simulink model "Twelve_quad_formation_301114"  (R2012b)
settings: Solver=ode5  StartTime=0.0  StopTime=inf  FixedStep=sample_time  RelTol=1e-3
InitFcn:
  | sample_time=0.005;%0.004;%0.0025;%0.02;
  | sample_time_Vicon = 0.005;
  | DeltaT = 0.02;
  | g = 9.81;
  | H0 = g%0.3165;
  | Kl = 1;
  | 
  | Q6_mass = 0.8;
  | 
  | Q6_Omega_r = 1.2; %for horizon ref
  | Q6_Zeta_r = 0.707; %for horizon ref
  | Q6_Omega_r_h = 2;%for vertical ref
  | Q6_Zeta_r_h = 0.7; %for vertical ref
  | 
  | 
  | Q6_Omega = 1.5; %for horizon control
  | Q6_Zeta = 0.507; %for horizon control
  | Q6_Omega_h= 2 %for vertical control
  | Q6_Zeta_h = 0.5; %for vertical control
  | 
  | 
  | Q6_acc_max = 5;%horizontal max acc
  | Q6_acc_max_h = 5;%horizontal max acc
  | 
  | omega_circle = 10*pi/180;
  | 
  | omega_h = 0.1;%Ascending speed
  | PI = pi;
  | Circle_R = 2;
  | 
  | 
  | MAX_Height = -2;
  | 
  | 
  | % for NN
  | n = 5;
  | r = 3;
  | n2 = 5;
  | NN_ST = 0.02;
  | 
  | GAMA_V = 6;
  | gama_V_e = 0.01;
  | 
  | GAMA_W = GAMA_V;
  | gama_W_e =0.01;
  | 
  | % deadzone
  | NN_Deadzone_Z = 0;
  | 
  | % inputs nomalizaton parameters
  | NN_Z_y_min = -3;
  | NN_Z_y_max = 0.5;
  | 
  | NN_Z_v_max = 8;
  | NN_Z_v_min = -NN_Z_v_max;
  | 
  | % alpha = 0.034;
  | alpha = 1;
  | % c_f = 0.0015;
  | c_f = 0.001;
  | ... (+1 lines)
libraries: X330_Control x60, simulink x24
(part 3 of 3)

== system Twelve_quad_formation_301114/Vicon_Data/Process Vicon Raw Data and Filter 8/Flip_pi1/Flip_0_to_2pi/Flip_2pi ==
  Angle : Inport
  Bias : Bias  Bias=-2*pi
  Constant : Constant  Value=2*pi
  Data Type Duplicate : DataTypeDuplicate
  Modulo : Math  Operator=mod  SaturateOnIntegerOverflow=on
  Sign1 : Signum
  Switch : Switch
  Angle_Flip : Outport
  wires:
  Angle/1 -> Modulo/1, Sign1/1, Data Type Duplicate/1
  Constant/1 -> Modulo/2
  Modulo/1 -> Bias/1, Switch/1
  Sign1/1 -> Switch/2
  Bias/1 -> Switch/3
  Switch/1 -> Angle_Flip/1, Data Type Duplicate/2

== system Twelve_quad_formation_301114/Vicon_Data/Process Vicon Raw Data and Filter 9/Flip_pi1/Flip_0_to_2pi/Flip_2pi ==
  Angle : Inport
  Bias : Bias  Bias=-2*pi
  Constant : Constant  Value=2*pi
  Data Type Duplicate : DataTypeDuplicate
  Modulo : Math  Operator=mod  SaturateOnIntegerOverflow=on
  Sign1 : Signum
  Switch : Switch
  Angle_Flip : Outport
  wires:
  Switch/1 -> Data Type Duplicate/2, Angle_Flip/1
  Bias/1 -> Switch/3
  Sign1/1 -> Switch/2
  Modulo/1 -> Switch/1, Bias/1
  Constant/1 -> Modulo/2
  Angle/1 -> Data Type Duplicate/1, Sign1/1, Modulo/1

== stateflow chart Twelve_quad_formation_301114/Subsystem/Trajectory Logic/ SF ==
  state Airborne
    state Stage6
      state Red_UAV1 [parallel]
        du:PosDes_UAV1[0] = (-1.457 - PosDes_UAV1[0])*0.5*DeltaT + PosDes_UAV1[0];
        PosDes_UAV1[1] = (1.457 - PosDes_UAV1[1])*0.5*DeltaT + PosDes_UAV1[1] ;
        PosDes_UAV1[2] = -1.2;
        settings: executionOrder=1
      state PWM1 [parallel]
        du:    Increm = Increm + DeltaT
        settings: executionOrder=2
      state Green_UAV2 [parallel]
        du:PosDes_UAV2[0] =(1.457 - PosDes_UAV2[0])*0.5*DeltaT + PosDes_UAV2[0] ;
        PosDes_UAV2[1] = (1.457 - PosDes_UAV2[1])*0.5*DeltaT + PosDes_UAV2[1];
        PosDes_UAV2[2] = -1.2;
        settings: executionOrder=3
      state Blue_UAV3 [parallel]
        du:PosDes_UAV3[0] = (-1.457 - PosDes_UAV3[0])*0.5*DeltaT + PosDes_UAV3[0] ;
        PosDes_UAV3[1] = (-1.457 - PosDes_UAV3[1])*0.5*DeltaT + PosDes_UAV3[1];
        PosDes_UAV3[2] = -1.2;
        settings: executionOrder=4
      state Purple_UAV4 [parallel]
        du:PosDes_UAV4[0] = (1.457 - PosDes_UAV4[0])*0.5*DeltaT + PosDes_UAV4[0];
        PosDes_UAV4[1] = (-1.457 - PosDes_UAV4[1])*0.5*DeltaT + PosDes_UAV4[1];
        PosDes_UAV4[2] = -1.2;
        settings: executionOrder=5
    state TakeOff
      du:		HoverThrottle = (H0 - HoverThrottle)*2*DeltaT + HoverThrottle ;
      PosDes_UAV1[2] = (-1.2 - PosDes_UAV1[2])*1*DeltaT + PosDes_UAV1[2] ; PosDes_UAV7[2] = (-1.2 - PosDes_UAV7[2])*1*DeltaT + PosDes_UAV7[2] ;
      PosDes_UAV2[2] = (-1.2 - PosDes_UAV2[2])*1*DeltaT + PosDes_UAV2[2] ; PosDes_UAV8[2] = (-1.2 - PosDes_UAV8[2])*1*DeltaT + PosDes_UAV8[2] ;
      PosDes_UAV3[2] = (-1.2 - PosDes_UAV3[2])*1*DeltaT + PosDes_UAV3[2] ; PosDes_UAV9[2] = (-1.2 - PosDes_UAV9[2])*1*DeltaT + PosDes_UAV9[2] ;
      PosDes_UAV4[2] = (-1.2 - PosDes_UAV4[2])*1*DeltaT + PosDes_UAV4[2] ; PosDes_UAV10[2] = (-1.2 - PosDes_UAV10[2])*1*DeltaT + PosDes_UAV10[2] ;
      PosDes_UAV5[2] = (-1.2 - PosDes_UAV5[2])*1*DeltaT + PosDes_UAV5[2] ; PosDes_UAV11[2] = (-1.2 - PosDes_UAV11[2])*1*DeltaT + PosDes_UAV11[2] ;
      PosDes_UAV6[2] = (-1.2 - PosDes_UAV6[2])*1*DeltaT + PosDes_UAV6[2] ; PosDes_UAV12[2] = (-1.2 - PosDes_UAV12[2])*1*DeltaT + PosDes_UAV12[2] ;
    state Stage1
      state Purple_UAV7 [parallel]
        du:PosDes_UAV7[0] = (3-PosDes_UAV7[0])*0.75*DeltaT + PosDes_UAV7[0];
        PosDes_UAV7[1] = (-1-PosDes_UAV7[1])*0.75*DeltaT+PosDes_UAV7[1];
        PosDes_UAV7[2] = (-1.2-PosDes_UAV7[2])*0.75*DeltaT+PosDes_UAV7[2];
        settings: executionOrder=1
      state Red_UAV1 [parallel]
        du:PosDes_UAV1[0] = (3- PosDes_UAV1[0])*0.75*DeltaT + PosDes_UAV1[0] ;
        PosDes_UAV1[1] = (3- PosDes_UAV1[1])*0.75*DeltaT + PosDes_UAV1[1] ;
        PosDes_UAV1[2] = (-1.2- PosDes_UAV1[2])*0.75*DeltaT + PosDes_UAV1[2] ;
        settings: executionOrder=2
      state Purple_UAV8 [parallel]
        du:PosDes_UAV8[0] = (-3-PosDes_UAV8[0])*0.75*DeltaT + PosDes_UAV8[0];
        PosDes_UAV8[1] = (-1-PosDes_UAV8[1])*0.75*DeltaT+PosDes_UAV8[1];
        PosDes_UAV8[2] = (-1.2-PosDes_UAV8[2])*0.75*DeltaT+PosDes_UAV8[2];
        settings: executionOrder=3
      state Green_UAV2 [parallel]
        du:PosDes_UAV2[0] = (-3-PosDes_UAV2[0])*0.75*DeltaT+PosDes_UAV2[0];
        PosDes_UAV2[1] = (3-PosDes_UAV2[1])*0.75*DeltaT+PosDes_UAV2[1];
        PosDes_UAV2[2] = (-1.2-PosDes_UAV2[2])*0.75*DeltaT+PosDes_UAV2[2];
        settings: executionOrder=4
      state Blue_UAV3 [parallel]
        du:PosDes_UAV3[0] = (3-PosDes_UAV3[0])*0.75*DeltaT + PosDes_UAV3[0];
        PosDes_UAV3[1] = (2-PosDes_UAV3[1])*0.75*DeltaT+PosDes_UAV3[1];
        PosDes_UAV3[2] = (-1.2-PosDes_UAV3[2])*0.75*DeltaT+PosDes_UAV3[2];
        settings: executionOrder=5
      state Purple_UAV9 [parallel]
        du:PosDes_UAV9[0] = (3-PosDes_UAV9[0])*0.75*DeltaT + PosDes_UAV9[0];
        PosDes_UAV9[1] = (-2-PosDes_UAV9[1])*0.75*DeltaT+PosDes_UAV9[1];
        PosDes_UAV9[2] = (-1.2-PosDes_UAV9[2])*0.75*DeltaT+PosDes_UAV9[2];
        settings: executionOrder=6
      state Purple_UAV4 [parallel]
        du:PosDes_UAV4[0] = (-3-PosDes_UAV4[0])*0.75*DeltaT + PosDes_UAV4[0];
        PosDes_UAV4[1] = (2-PosDes_UAV4[1])*0.75*DeltaT+PosDes_UAV4[1];
        PosDes_UAV4[2] = (-1.2-PosDes_UAV4[2])*0.75*DeltaT+PosDes_UAV4[2];
        settings: executionOrder=7
      state Purple_UAV12 [parallel]
        du:PosDes_UAV10[0] = (-3-PosDes_UAV10[0])*0.75*DeltaT + PosDes_UAV10[0];
        PosDes_UAV10[1] = (-2-PosDes_UAV10[1])*0.75*DeltaT+PosDes_UAV10[1];
        PosDes_UAV10[2] = (-1.2-PosDes_UAV10[2])*0.75*DeltaT+PosDes_UAV10[2];
        settings: executionOrder=8
      state Purple_UAV5 [parallel]
        du:PosDes_UAV5[0] = (3-PosDes_UAV5[0])*0.75*DeltaT + PosDes_UAV5[0];
        PosDes_UAV5[1] = (1-PosDes_UAV5[1])*0.75*DeltaT+PosDes_UAV5[1];
        PosDes_UAV5[2] = (-1.2-PosDes_UAV5[2])*0.75*DeltaT+PosDes_UAV5[2];
        settings: executionOrder=9
      state Purple_UAV11 [parallel]
        du:PosDes_UAV11[0] = (3-PosDes_UAV11[0])*0.75*DeltaT + PosDes_UAV11[0];
        PosDes_UAV11[1] = (-3-PosDes_UAV11[1])*0.75*DeltaT+PosDes_UAV11[1];
        PosDes_UAV11[2] = (-1.2-PosDes_UAV11[2])*0.75*DeltaT+PosDes_UAV11[2];
        settings: executionOrder=10
      state Purple_UAV6 [parallel]
        du:PosDes_UAV6[0] = (-3-PosDes_UAV6[0])*0.75*DeltaT + PosDes_UAV6[0];
        PosDes_UAV6[1] = (1-PosDes_UAV6[1])*0.75*DeltaT+PosDes_UAV6[1];
        PosDes_UAV6[2] = (-1.2-PosDes_UAV6[2])*0.75*DeltaT+PosDes_UAV6[2];
        settings: executionOrder=11
      state Purple_UAV10 [parallel]
        du:PosDes_UAV4[0] = (-3-PosDes_UAV4[0])*0.75*DeltaT + PosDes_UAV4[0];
        PosDes_UAV4[1] = (-3-PosDes_UAV4[1])*0.75*DeltaT+PosDes_UAV4[1];
        PosDes_UAV4[2] = (-1.2-PosDes_UAV4[2])*0.75*DeltaT+PosDes_UAV4[2];
        settings: executionOrder=12
    state Stage7
      state Red_UAV1 [parallel]
        du:PosDes_UAV1[0] = 3.5*cos(81.087*PI/180-Increm*omega_circle)-2;
        PosDes_UAV1[1] = 3.5*sin(81.087*PI/180-Increm*omega_circle)-2 ;
        PosDes_UAV1[2] = -1.2;
        settings: executionOrder=1
      state PWM1 [parallel]
        du:    Increm = Increm + DeltaT
        settings: executionOrder=2
      state Green_UAV2 [parallel]
        du:PosDes_UAV2[0] = 3.5*cos(351.087*PI/180-Increm*omega_circle)-2;
        PosDes_UAV2[1] = 3.5*sin(351.087*PI/180-Increm*omega_circle)+2;
        PosDes_UAV2[2] = -1.2;
        settings: executionOrder=3
      state Blue_UAV3 [parallel]
        du:PosDes_UAV3[0] = 3.5*cos(171.087*PI/180-Increm*omega_circle)+2  ;
        PosDes_UAV3[1] = 3.5*sin(171.087*PI/180-Increm*omega_circle)-2;
        PosDes_UAV3[2] = -1.2;
        settings: executionOrder=4
      state Purple_UAV4 [parallel]
        du:PosDes_UAV4[0] = 3.5*cos(261.087*PI/180-Increm*omega_circle)+2 ;
        PosDes_UAV4[1] = 3.5*sin(261.087*PI/180-Increm*omega_circle)+2;
        PosDes_UAV4[2] = -1.2;
        settings: executionOrder=5
    state Stage2
      state Red_UAV1 [parallel]
        du:PosDes_UAV1[0] = (0.8 - PosDes_UAV1[0])*0.5*DeltaT + PosDes_UAV1[0]  ;
        PosDes_UAV1[1] = (2 - PosDes_UAV1[1])*0.5*DeltaT + PosDes_UAV1[1]  ;
        PosDes_UAV1[2] = -1.2 ;
        settings: executionOrder=1
      state PWM2 [parallel]
        du:    Increm = Increm + DeltaT
        settings: executionOrder=2
      state Green_UAV2 [parallel]
        du:PosDes_UAV2[0] = (-0.8 - PosDes_UAV2[0])*0.5*DeltaT + PosDes_UAV2[0];
        PosDes_UAV2[1] = (2 - PosDes_UAV2[1])*0.5*DeltaT + PosDes_UAV2[1];
        PosDes_UAV2[2] = -1.2;
        settings: executionOrder=3
      state Blue_UAV3 [parallel]
        du:PosDes_UAV3[0] = (0.8 - PosDes_UAV3[0])*0.5*DeltaT + PosDes_UAV3[0];
        PosDes_UAV3[1] = (-2 - PosDes_UAV3[1])*0.5*DeltaT + PosDes_UAV3[1];
        PosDes_UAV3[2] = -1.2;
        settings: executionOrder=4
      state Purple_UAV4 [parallel]
        du:PosDes_UAV4[0] = (-0.8 - PosDes_UAV4[0])*0.5*DeltaT + PosDes_UAV4[0];
        PosDes_UAV4[1] = (-2 - PosDes_UAV4[1])*0.5*DeltaT + PosDes_UAV4[1];
        PosDes_UAV4[2] = -1.2;
        settings: executionOrder=5
    state Stage8
      state Red_UAV1 [parallel]
        du:PosDes_UAV1[0] = (2 - PosDes_UAV1[0])*0.5*DeltaT + PosDes_UAV1[0];
        PosDes_UAV1[1] = (-2 - PosDes_UAV1[1])*0.5*DeltaT + PosDes_UAV1[1];
        PosDes_UAV1[2] = -1.2;
        settings: executionOrder=1
      state PWM1 [parallel]
        du:    Increm = Increm + DeltaT
        settings: executionOrder=2
      state Green_UAV2 [parallel]
        du:PosDes_UAV2[0] = (-2 - PosDes_UAV2[0])*0.5*DeltaT + PosDes_UAV2[0];
        PosDes_UAV2[1] = (-2 - PosDes_UAV2[1])*0.5*DeltaT + PosDes_UAV2[1];
        PosDes_UAV2[2] = -1.2;
        settings: executionOrder=3
      state Blue_UAV3 [parallel]
        du:PosDes_UAV3[0] = (2 - PosDes_UAV3[0])*0.5*DeltaT + PosDes_UAV3[0] ;
        PosDes_UAV3[1] = (2 - PosDes_UAV3[1])*0.5*DeltaT + PosDes_UAV3[1];
        PosDes_UAV3[2] = -1.2;
        settings: executionOrder=4
      state Purple_UAV4 [parallel]
        du:PosDes_UAV4[0] = (-2 - PosDes_UAV4[0])*0.5*DeltaT + PosDes_UAV4[0];
        PosDes_UAV4[1] = (2 - PosDes_UAV4[1])*0.5*DeltaT + PosDes_UAV4[1];
        PosDes_UAV4[2] = -1.2;
        settings: executionOrder=5
    state Stage3
      state Red_UAV1 [parallel]
        du:PosDes_UAV1[0] = 0.8-Increm;
        PosDes_UAV1[1] = 0.625*(0.8-Increm)*(0.8-Increm)+1.6 ;
        PosDes_UAV1[2] = -1.2;
        settings: executionOrder=1
      state PWM1 [parallel]
        du:    Increm = Increm + DeltaT
        settings: executionOrder=2
      state Green_UAV2 [parallel]
        du:PosDes_UAV2[0] = -0.8+Increm;
        PosDes_UAV2[1] = -0.625*(0.8-Increm)*(0.8-Increm)+2.4;
        PosDes_UAV2[2] = -1.2;
        settings: executionOrder=3
      state Blue_UAV3 [parallel]
        du:PosDes_UAV3[0] = 0.8 - Increm;
        PosDes_UAV3[1] = 0.625*(0.8-Increm)*(0.8-Increm)-2.4;
        PosDes_UAV3[2] = -1.2;
        settings: executionOrder=4
      state Purple_UAV4 [parallel]
        du:PosDes_UAV4[0] = -0.8 + Increm;
        PosDes_UAV4[1] = -0.625*(0.8-Increm)*(0.8-Increm)-1.6;
        PosDes_UAV4[2] = -1.2;
        settings: executionOrder=5
    state Stage9
      state Red_UAV1 [parallel]
        du:PosDes_UAV1[0] = (0 - PosDes_UAV1[0])*0.5*DeltaT + PosDes_UAV1[0];
        PosDes_UAV1[1] = (-2 - PosDes_UAV1[1])*0.5*DeltaT + PosDes_UAV1[1];
        PosDes_UAV1[2] = -1.2;
        settings: executionOrder=1
      state PWM1 [parallel]
        du:    Increm = Increm + DeltaT
        settings: executionOrder=2
      state Green_UAV2 [parallel]
        du:PosDes_UAV2[0] = (0 - PosDes_UAV2[0])*0.5*DeltaT + PosDes_UAV2[0];
        PosDes_UAV2[1] = (-0.667 - PosDes_UAV2[1])*0.5*DeltaT + PosDes_UAV2[1];
        PosDes_UAV2[2] = -1.2;
        settings: executionOrder=3
      state Blue_UAV3 [parallel]
        du:PosDes_UAV3[0] = (0 - PosDes_UAV3[0])*0.5*DeltaT + PosDes_UAV3[0] ;
        PosDes_UAV3[1] = (0.667 - PosDes_UAV3[1])*0.5*DeltaT + PosDes_UAV3[1];
        PosDes_UAV3[2] = -1.2;
        settings: executionOrder=4
      state Purple_UAV4 [parallel]
        du:PosDes_UAV4[0] = (0 - PosDes_UAV4[0])*0.5*DeltaT + PosDes_UAV4[0];
        PosDes_UAV4[1] = (2 - PosDes_UAV4[1])*0.5*DeltaT + PosDes_UAV4[1];
        PosDes_UAV4[2] = -1.2;
        settings: executionOrder=5
    state Stage4
      state Red_UAV1 [parallel]
        du:PosDes_UAV1[0] = (-2 - PosDes_UAV1[0])*0.5*DeltaT + PosDes_UAV1[0];
        PosDes_UAV1[1] = (2 - PosDes_UAV1[1])*0.5*DeltaT + PosDes_UAV1[1] ;
        PosDes_UAV1[2] = -1.2;
        settings: executionOrder=1
      state PWM1 [parallel]
        du:    Increm = Increm + DeltaT
        settings: executionOrder=2
      state Green_UAV2 [parallel]
        du:PosDes_UAV2[0] = (2 - PosDes_UAV2[0])*0.5*DeltaT + PosDes_UAV2[0];
        PosDes_UAV2[1] = (2 - PosDes_UAV2[1])*0.5*DeltaT + PosDes_UAV2[1];
        PosDes_UAV2[2] = -1.2;
        settings: executionOrder=3
      state Blue_UAV3 [parallel]
        du:PosDes_UAV3[0] = (-2 - PosDes_UAV3[0])*0.5*DeltaT + PosDes_UAV3[0]  ;
        PosDes_UAV3[1] = (-2 - PosDes_UAV3[1])*0.5*DeltaT + PosDes_UAV3[1];
        PosDes_UAV3[2] = -1.2;
        settings: executionOrder=4
      state Purple_UAV4 [parallel]
        du:PosDes_UAV4[0] = (2- PosDes_UAV4[0])*0.5*DeltaT + PosDes_UAV4[0];
        PosDes_UAV4[1] = (-2 - PosDes_UAV4[1])*0.5*DeltaT + PosDes_UAV4[1];
        PosDes_UAV4[2] = -1.2;
        settings: executionOrder=5
    state Stage10
      state Red_UAV1 [parallel]
        du:PosDes_UAV1[0] = 2*sin(180*PI/180-Increm*omega_circle);
        PosDes_UAV1[1] =  2*cos(180*PI/180-Increm*omega_circle);
        PosDes_UAV1[2] = -1.2;
        settings: executionOrder=1
      state PWM1 [parallel]
        du:    Increm = Increm + DeltaT
        settings: executionOrder=2
      state Green_UAV2 [parallel]
        du:PosDes_UAV2[0] = 0.667*sin(180*PI/180-Increm*omega_circle);
        PosDes_UAV2[1] = 0.667*cos(180*PI/180-Increm*omega_circle);
        PosDes_UAV2[2] = -1.2;
        settings: executionOrder=3
      state Blue_UAV3 [parallel]
        du:PosDes_UAV3[0] = 0.667*sin(0*PI/180-Increm*omega_circle) ;
        PosDes_UAV3[1] = 0.667*cos(0*PI/180-Increm*omega_circle);
        PosDes_UAV3[2] = -1.2;
        settings: executionOrder=4
      state Purple_UAV4 [parallel]
        du:PosDes_UAV4[0] = 2*sin(0*PI/180-Increm*omega_circle);
        PosDes_UAV4[1] = 2*cos(0*PI/180-Increm*omega_circle);
        PosDes_UAV4[2] = -1.2;
        settings: executionOrder=5
    state Stage11
      state Red_UAV1 [parallel]
        du:PosDes_UAV1[0] = 2;
        PosDes_UAV1[1] = 0;
        PosDes_UAV1[2] = -1.2;
        settings: executionOrder=1
      state Green_UAV2 [parallel]
        du:PosDes_UAV2[0] = 0.75;
        PosDes_UAV2[1] = 0;
        PosDes_UAV2[2] = -1.2;
        settings: executionOrder=2
      state Blue_UAV3 [parallel]
        du:PosDes_UAV3[0] = -0.75 ;
        PosDes_UAV3[1] = 0;
        PosDes_UAV3[2] = -1.2;
        settings: executionOrder=3
      state Purple_UAV4 [parallel]
        du:PosDes_UAV4[0] = -2;
        PosDes_UAV4[1] = 0;
        PosDes_UAV4[2] = -1.2;
        settings: executionOrder=4
    state Stage5
      state Red_UAV1 [parallel]
        du:PosDes_UAV1[0] = -2;
        PosDes_UAV1[1] = 2 ;
        PosDes_UAV1[2] = -1.2;
        settings: executionOrder=1
      state PWM1 [parallel]
        du:    Increm = Increm + DeltaT
        settings: executionOrder=2
      state Green_UAV2 [parallel]
        du:PosDes_UAV2[0] = 2 ;
        PosDes_UAV2[1] = 2;
        PosDes_UAV2[2] = -1.2;
        settings: executionOrder=3
      state Blue_UAV3 [parallel]
        du:PosDes_UAV3[0] = -2  ;
        PosDes_UAV3[1] = -2;
        PosDes_UAV3[2] = -1.2;
        settings: executionOrder=4
      state Purple_UAV4 [parallel]
        du:PosDes_UAV4[0] = 2 ;
        PosDes_UAV4[1] = -2;
        PosDes_UAV4[2] = -1.2;
        settings: executionOrder=5
    (default) -> TakeOff : {	PosDes_UAV1 = Pos_UAV1;
        | 	PosDes_UAV2 = Pos_UAV2;
        | 	PosDes_UAV3 = Pos_UAV3;
        | 	PosDes_UAV4 = Pos_UAV4;
        | 	 }
    Stage5 -> Stage6 : after(3,sec)
    TakeOff -> Stage1 : after (3, sec)
    Stage6 -> Stage7 : [(abs(Pos_UAV1[0]-(-1.457)))<0.2]
        | {Increm = 0;}
    Stage1 -> Stage2 : after (3, sec)
        | {Increm =0;}
    Stage7 -> Stage8 : [(abs(Pos_UAV1[0]-1.457))<0.2]
        | {Increm = 0;}
    Stage2 -> Stage3 : [(abs(Pos_UAV1[0]-0.8))<0.2]
        | {Increm = 0;}
    Stage8 -> Stage9 : after (3,sec)
        | {Increm = 0;}
    Stage3 -> Stage4 : [(abs(Pos_UAV1[0]-(-0.8)))<0.2]
        | {Increm = 0;}
    Stage9 -> Stage10 : after (5, sec)
        | {Increm =0;}
    Stage4 -> Stage5 : [(abs(Pos_UAV1[0]-(-2)))<0.2]
        | {Increm = 0;}
    Stage10 -> Stage11 : [(abs(Pos_UAV1[0]-2))<0.1]
  state Landing
    state Decsending
      en:		PosDes_UAV1 = Pos_UAV1;	PosDes_UAV2 = Pos_UAV2;  PosDes_UAV3 = Pos_UAV3;
      PosDes_UAV4 = Pos_UAV4; PosDes_UAV5 = Pos_UAV5; PosDes_UAV6 = Pos_UAV6;
      PosDes_UAV7 = Pos_UAV7; PosDes_UAV8 = Pos_UAV8; PosDes_UAV9 = Pos_UAV9;
      PosDes_UAV10 = Pos_UAV10; PosDes_UAV11 = Pos_UAV11; PosDes_UAV12 = Pos_UAV12;
      du:		PosDes_UAV1[2] = (0 - PosDes_UAV1[2])*0.2*DeltaT + PosDes_UAV1[2] ;
      PosDes_UAV2[2] = (0 - PosDes_UAV2[2])*0.2*DeltaT + PosDes_UAV2[2] ;
      PosDes_UAV3[2] = (0 - PosDes_UAV3[2])*0.2*DeltaT + PosDes_UAV3[2] ;
      PosDes_UAV4[2] = (0 - PosDes_UAV4[2])*0.2*DeltaT + PosDes_UAV4[2] ;
      PosDes_UAV5[2] = (0 - PosDes_UAV5[2])*0.2*DeltaT + PosDes_UAV5[2] ;
      PosDes_UAV6[2] = (0 - PosDes_UAV6[2])*0.2*DeltaT + PosDes_UAV6[2] ;
      PosDes_UAV7[2] = (0 - PosDes_UAV7[2])*0.2*DeltaT + PosDes_UAV7[2] ;
      PosDes_UAV8[2] = (0 - PosDes_UAV8[2])*0.2*DeltaT + PosDes_UAV8[2] ;
      PosDes_UAV9[2] = (0 - PosDes_UAV9[2])*0.2*DeltaT + PosDes_UAV9[2] ;
      PosDes_UAV10[2] = (0 - PosDes_UAV10[2])*0.2*DeltaT + PosDes_UAV10[2] ;
      PosDes_UAV11[2] = (0 - PosDes_UAV11[2])*0.2*DeltaT + PosDes_UAV11[2] ;
      PosDes_UAV12[2] = (0 - PosDes_UAV12[2])*0.2*DeltaT + PosDes_UAV12[2] ;
    state CutThrottle
      du:		HoverThrottle = (0.0 - HoverThrottle)*3*DeltaT + HoverThrottle ;
    (default) -> Decsending
    Decsending -> (junction 288) : after(2,sec)
    (junction 288) -> CutThrottle : [Pos_UAV1[2] > -0.2]
  Landing -> Airborne : [RC[6] > 0.5]
  Airborne -> Landing : [RC[6] < -0.5]
  (default) -> Landing : {HoverThrottle=0.0}
  data: HoverThrottle output double size=1; PosDes_UAV1 output double size=4; PosDes_UAV2 output double size=4; PosDes_UAV3 output double size=4; RC input size=8; Pos_UAV1 input size=4; DeltaT parameter size=1; H0 parameter size=1; Kl parameter size=1; Increm local double size=1; omega_circle parameter size=1; PI parameter size=1; omega_h parameter; Circle_R parameter size=1; MAX_Height parameter size=1; Pos_UAV2 input size=4; Pos_UAV3 input size=4; Pos_UAV4 input size=4; PosDes_UAV4 output double size=4; Pos_UAV5 input size=4; Pos_UAV6 input size=4; Pos_UAV7 input size=4; Pos_UAV8 input size=4; Pos_UAV9 input size=4; Pos_UAV10 input size=4; Pos_UAV11 input size=4; Pos_UAV12 input size=4; PosDes_UAV5 output double size=4; PosDes_UAV6 output double size=4; PosDes_UAV7 output double size=4; PosDes_UAV8 output double size=4; PosDes_UAV9 output double size=4; PosDes_UAV10 output double size=4; PosDes_UAV11 output double size=4; PosDes_UAV12 output double size=4
